simulink model "snb_a"  (R2012b)
settings: Solver=FixedStepDiscrete  SolverMode=SingleTasking  StartTime=0.0  StopTime=10000  RelTol=1e-3
undefined symbols (not defined in the file): Down, Up
libraries: xbsIndex_r4 x9360, casper_library_misc x16, casper_library_communications x8, xps_library x4, casper_library_delays x2
(part 5 of 71)

== system snb_a/coarse_delay3 ==
  note: new delay values/enables come aligned
      | with data, need to be one cycle before
      | so new delay value gets loaded at the
      | same time as data, so delay data path
      | by one cycle
  sync_in : Inport
  din0 : Inport  Port=2
  en : Inport  Port=3
  delay_val0 : Inport  Port=4
  load_val0 : Inport  Port=5
  Concat4 : xbsIndex_r4/Concat  num_inputs=8  dbl_ovrd=off  block_type=concat
  Delay36 : xbsIndex_r4/Delay  rst=off  infoeditControl=Selection of Reset will increase slice count due to use of real FFs and instead of SRLs  en=off  latency=1  dbl_ovrd=off  reg_retiming=on  block_type=delay
  Delay37 : xbsIndex_r4/Delay  rst=off  infoeditControl=Selection of Reset will increase slice count due to use of real FFs and instead of SRLs  en=off  latency=1  dbl_ovrd=off  reg_retiming=on  block_type=delay
  Delay38 : xbsIndex_r4/Delay  rst=off  infoeditControl=Selection of Reset will increase slice count due to use of real FFs and instead of SRLs  en=off  latency=1  dbl_ovrd=off  reg_retiming=on  block_type=delay
  Reinterpret{,1..7} (8 alike) : xbsIndex_r4/Reinterpret  force_arith_type=on  arith_type=Unsigned  force_bin_pt=on  bin_pt=0  block_type=reinterpret
  Terminator34 : Terminator
  Terminator38 : Terminator
  Terminator39 : Terminator
  bus_expand14 : Subsystem  AncestorBlock=casper_library_flow_control/bus_expand  mask(bus_expand){mode=divisions of arbitrary size, outputNum=1, outputWidth=[16+15 16 16 16], outputBinaryPt=[16 15 15 15], outputArithmeticType=[0 1 1 1], show_format=off, outputToWorkspace=off, variablePrefix=out, outputToModelAsWell=on}
      mask prompts: outputNum "Number of outputs:"; outputWidth "Output width [msb ... lsb]:"; outputBinaryPt "Output binary point position [msb ... lsb]:"; outputArithmeticType "Output arithmetic type (ufix=0, fix=1, bool=2) [msb ... lsb]:"; show_format "Print format string?"; outputToWorkspace "Output to workspace?"; variablePrefix "Variable name prefix:"; outputToModelAsWell "Output to model as well?"
      mask help:
      | Expands a 'bus' made using a bus_create or Xilinx
      | concat block.
      | The input will be divided into the specified number
      | of outputs with the specified arithmetic types.
      | Divisions are made from most significant bit.
      mask init: same as snb_a/bus_expand10
      settings: AttributesFormatString=4 outputs
      mask TypeOptions mode: divisions of equal size | divisions of arbitrary size
      mask Callback mode: bus_expand_callback();
      mask Callback outputWidth: bus_expand_callback();
      mask Callback outputToWorkspace: bus_expand_callback();
  bus_expand7 : Subsystem  AncestorBlock=casper_library_flow_control/bus_expand  mask(bus_expand){mode=divisions of equal size, outputNum=8, outputWidth=10, outputBinaryPt=9, outputArithmeticType=1, show_format=off, outputToWorkspace=off, variablePrefix=out, outputToModelAsWell=on}
      mask prompts: outputNum "Number of outputs:"; outputWidth "Output width:"; outputBinaryPt "Output binary point position:"; outputArithmeticType "Output arithmetic type (ufix=0, fix=1, bool=2):"; show_format "Print format string?"; outputToWorkspace "Output to workspace?"; variablePrefix "Variable name prefix:"; outputToModelAsWell "Output to model as well?"
      mask help:
      | Expands a 'bus' made using a bus_create or Xilinx
      | concat block.
      | The input will be divided into the specified number
      | of outputs with the specified arithmetic types.
      | Divisions are made from most significant bit.
      mask init: same as snb_a/bus_expand10
      settings: AttributesFormatString=8 outputs
      mask TypeOptions mode: divisions of equal size | divisions of arbitrary size
      mask Callback mode: bus_expand_callback();
      mask Callback outputWidth: bus_expand_callback();
      mask Callback outputToWorkspace: bus_expand_callback();
  delay_gen0 : Subsystem  mask{n_bits_fft_words=10, n_bits_streams=3, n_bits_fft=12, n_bits_data=10}
      mask prompts: n_bits_fft_words "FFT size (2^? data words)"; n_bits_streams "parallel data streams (2^?)"; n_bits_fft "effective FFT size (2^? bins)"; n_bits_data "data bit width"
  delay_wideband_prog0 : Subsystem  AncestorBlock=casper_library_delays/delay_wideband_prog  mask(delay_wideband_prog){max_delay=8192, n_inputs_bits=3, bram_latency=2, bram_type=Dual Port, async=on}
      mask prompts: max_delay "Max Delay (Sample Clks)"; n_inputs_bits "Number of Simultaneous Inputs(2^?)"; bram_latency "BRAM Latency"; bram_type "Select type of BRAM"; async "asynchronous operation"
      mask init:
      | delay_wideband_prog_init(gcb,...
      |     'max_delay',max_delay,...
      |     'n_inputs_bits',n_inputs_bits,...
      |     'bram_latency',bram_latency,...
      |     'bram_type',bram_type, ...
      |     'async', async);
      mask TypeOptions bram_type: Single Port | Dual Port
  sync_out : Outport
  dout0 : Outport  Port=2
  dvalid : Outport  Port=3
  wires:
  Reinterpret7/1 -> Concat4/8
  Reinterpret6/1 -> Concat4/7
  Reinterpret4/1 -> Concat4/5
  Reinterpret5/1 -> Concat4/6
  Reinterpret3/1 -> Concat4/4
  Reinterpret2/1 -> Concat4/3
  Reinterpret1/1 -> Concat4/2
  Reinterpret/1 -> Concat4/1
  delay_gen0/6(slope) -> Terminator39/1
  delay_gen0/5(initial_phase) -> Terminator38/1
  delay_gen0/3(idx_out) -> Terminator34/1
  din0/1 -> delay_gen0/2(din)
  bus_expand14/4(lsb_out1) -> delay_gen0/7(d/dt_phase)
  bus_expand14/3(out2) -> delay_gen0/6(phase)
  bus_expand14/2(out3) -> delay_gen0/5(d/dt_delay)
  bus_expand14/1(msb_out4) -> delay_gen0/4(delay)
  sync_in/1 -> delay_gen0/1(sync_in)
  delay_gen0/4(dvalid) -> Delay37/1
  delay_gen0/1(sync_out) -> Delay36/1
  delay_gen0/2(dout) -> Delay38/1
  delay_wideband_prog0/10(dvalid) -> dvalid/1
  bus_expand7/8(lsb_out1) -> delay_wideband_prog0/11(data_in7)
  bus_expand7/7(out2) -> delay_wideband_prog0/10(data_in6)
  bus_expand7/6(out3) -> delay_wideband_prog0/9(data_in5)
  bus_expand7/5(out4) -> delay_wideband_prog0/8(data_in4)
  bus_expand7/4(out5) -> delay_wideband_prog0/7(data_in3)
  bus_expand7/3(out6) -> delay_wideband_prog0/6(data_in2)
  bus_expand7/2(out7) -> delay_wideband_prog0/5(data_in1)
  bus_expand7/1(msb_out8) -> delay_wideband_prog0/4(data_in0)
  delay_gen0/8(new_value) -> delay_wideband_prog0/3(ld_delay)
  delay_gen0/7(coarse_delay) -> delay_wideband_prog0/2(delay)
  en/1 -> delay_gen0/3(en)
  load_val0/1 -> delay_gen0/8(ld)
  delay_val0/1 -> bus_expand14/1(bus_in)
  delay_wideband_prog0/1(sync_out) -> sync_out/1
  Delay38/1 -> bus_expand7/1(bus_in)
  delay_wideband_prog0/9(data_out7) -> Reinterpret7/1
  Delay36/1 -> delay_wideband_prog0/1(sync)
  delay_wideband_prog0/5(data_out3) -> Reinterpret3/1
  delay_wideband_prog0/4(data_out2) -> Reinterpret2/1
  Delay37/1 -> delay_wideband_prog0/12(en)
  Concat4/1 -> dout0/1
  delay_wideband_prog0/7(data_out5) -> Reinterpret5/1
  delay_wideband_prog0/8(data_out6) -> Reinterpret6/1
  delay_wideband_prog0/3(data_out1) -> Reinterpret1/1
  delay_wideband_prog0/6(data_out4) -> Reinterpret4/1
  delay_wideband_prog0/2(data_out0) -> Reinterpret/1

== system snb_a/control ==
  convert1_{1..21} (21 alike) : DataTypeConversion  OutDataTypeStr=fixdt('ufix1_En0')  LockScale=on
  convert2_{1..21} (21 alike) : DataTypeConversion  OutDataTypeStr=fixdt('ufix1_En0')  ConvertRealWorld=Stored Integer (SI)  LockScale=on
  gain_1 : Gain  Gain=1048576
  gain_10 : Gain  Gain=2048
  gain_11 : Gain  Gain=1024
  gain_12 : Gain  Gain=512
  gain_13 : Gain  Gain=256
  gain_14 : Gain  Gain=128
  gain_15 : Gain  Gain=64
  gain_16 : Gain  Gain=32
  gain_17 : Gain  Gain=16
  gain_18 : Gain  Gain=8
  gain_19 : Gain  Gain=4
  gain_2 : Gain  Gain=524288
  gain_20 : Gain  Gain=2
  gain_21 : Gain
  gain_3 : Gain  Gain=262144
  gain_4 : Gain  Gain=131072
  gain_5 : Gain  Gain=65536
  gain_6 : Gain  Gain=32768
  gain_7 : Gain  Gain=16384
  gain_8 : Gain  Gain=8192
  gain_9 : Gain  Gain=4096
  io_delay : xbsIndex_r4/Delay  rst=off  infoeditControl=Selection of Reset will increase slice count due to use of real FFs and instead of SRLs  en=off  latency=1  dbl_ovrd=off  reg_retiming=on  block_type=delay
  sim_{1..21} (21 alike) : Constant  Value=0
  sim_add : Sum  Inputs=+++++++++++++++++++++  OutDataTypeStr=uint32
  slice_adc_bad_clr : xbsIndex_r4/Slice  nbits=1  boolean_output=on  mode=Lower Bit Location + Width  bit1=0  base1=MSB of Input  bit0=15  base0=LSB of Input  dbl_ovrd=off  block_type=slice
  slice_adc_protect_disable : xbsIndex_r4/Slice  nbits=1  boolean_output=on  mode=Lower Bit Location + Width  bit1=0  base1=MSB of Input  bit0=14  base0=LSB of Input  dbl_ovrd=off  block_type=slice
  slice_arm : xbsIndex_r4/Slice  nbits=1  boolean_output=on  mode=Lower Bit Location + Width  bit1=0  base1=MSB of Input  bit0=19  base0=LSB of Input  dbl_ovrd=off  block_type=slice
  slice_cnt_rst : xbsIndex_r4/Slice  nbits=1  boolean_output=on  mode=Lower Bit Location + Width  bit1=0  base1=MSB of Input  bit0=8  base0=LSB of Input  dbl_ovrd=off  block_type=slice
  slice_gbe_cnt_rst : xbsIndex_r4/Slice  nbits=1  boolean_output=on  mode=Lower Bit Location + Width  bit1=0  base1=MSB of Input  bit0=7  base0=LSB of Input  dbl_ovrd=off  block_type=slice
  slice_gbe_rst : xbsIndex_r4/Slice  nbits=1  boolean_output=on  mode=Lower Bit Location + Width  bit1=0  base1=MSB of Input  bit0=17  base0=LSB of Input  dbl_ovrd=off  block_type=slice
  slice_gbe_txen : xbsIndex_r4/Slice  nbits=1  boolean_output=on  mode=Lower Bit Location + Width  bit1=0  base1=MSB of Input  bit0=16  base0=LSB of Input  dbl_ovrd=off  block_type=slice
  slice_snapcoarse_arm : xbsIndex_r4/Slice  nbits=1  boolean_output=on  mode=Lower Bit Location + Width  bit1=0  base1=MSB of Input  bit0=5  base0=LSB of Input  dbl_ovrd=off  block_type=slice
  slice_snappfb_arm : xbsIndex_r4/Slice  nbits=1  boolean_output=on  mode=Lower Bit Location + Width  bit1=0  base1=MSB of Input  bit0=4  base0=LSB of Input  dbl_ovrd=off  block_type=slice
  slice_snappfb_dsel : xbsIndex_r4/Slice  nbits=1  boolean_output=on  mode=Lower Bit Location + Width  bit1=0  base1=MSB of Input  bit0=3  base0=LSB of Input  dbl_ovrd=off  block_type=slice
  slice_snapquant_arm : xbsIndex_r4/Slice  nbits=1  boolean_output=on  mode=Lower Bit Location + Width  bit1=0  base1=MSB of Input  bit0=2  base0=LSB of Input  dbl_ovrd=off  block_type=slice
  slice_status_clr : xbsIndex_r4/Slice  nbits=1  boolean_output=on  mode=Lower Bit Location + Width  bit1=0  base1=MSB of Input  bit0=18  base0=LSB of Input  dbl_ovrd=off  block_type=slice
  slice_sys_rst : xbsIndex_r4/Slice  nbits=1  boolean_output=on  mode=Lower Bit Location + Width  bit1=0  base1=MSB of Input  bit0=20  base0=LSB of Input  dbl_ovrd=off  block_type=slice
  slice_tvg_adc : xbsIndex_r4/Slice  nbits=1  boolean_output=on  mode=Lower Bit Location + Width  bit1=0  base1=MSB of Input  bit0=9  base0=LSB of Input  dbl_ovrd=off  block_type=slice
  slice_tvg_ct : xbsIndex_r4/Slice  nbits=1  boolean_output=on  mode=Lower Bit Location + Width  bit1=0  base1=MSB of Input  bit0=12  base0=LSB of Input  dbl_ovrd=off  block_type=slice
  slice_tvg_d80 : xbsIndex_r4/Slice  nbits=1  boolean_output=on  mode=Lower Bit Location + Width  bit1=0  base1=MSB of Input  bit0=1  base0=LSB of Input  dbl_ovrd=off  block_type=slice
  slice_tvg_en : xbsIndex_r4/Slice  nbits=1  boolean_output=on  mode=Lower Bit Location + Width  bit1=0  base1=MSB of Input  bit0=13  base0=LSB of Input  dbl_ovrd=off  block_type=slice
  slice_tvg_fdfs : xbsIndex_r4/Slice  nbits=1  boolean_output=on  mode=Lower Bit Location + Width  bit1=0  base1=MSB of Input  bit0=10  base0=LSB of Input  dbl_ovrd=off  block_type=slice
  slice_tvg_packetiser : xbsIndex_r4/Slice  nbits=1  boolean_output=on  mode=Lower Bit Location + Width  bit1=0  base1=MSB of Input  bit0=11  base0=LSB of Input  dbl_ovrd=off  block_type=slice
  slice_unpack_cnt_rst : xbsIndex_r4/Slice  nbits=1  boolean_output=on  mode=Lower Bit Location + Width  bit1=0  base1=MSB of Input  bit0=6  base0=LSB of Input  dbl_ovrd=off  block_type=slice
  slice_wintime_snap_wesel : xbsIndex_r4/Slice  nbits=1  boolean_output=on  mode=Lower Bit Location + Width  bit1=0  base1=MSB of Input  bit0=0  base0=LSB of Input  dbl_ovrd=off  block_type=slice
  snb_a_control_user_data_out : xbsIndex_r4/Gateway In  gui_display_data_type=Fixed-point  arith_type=Unsigned  n_bits=32  bin_pt=0  preci_type=Single  exp_width=8  frac_width=24  quantization="Round  (unbiased: +/- Inf)"  overflow=Saturate  period=1  dbl_ovrd=off  timing_constraint=None  locs_specified=off  LOCs={}  UseAsADC=off  ADCChannel='1'  inherit_from_input=off  hdl_port=on  block_type=gatewayin
  in_sys_rst : Outport
  in_arm : Outport  Port=2
  in_status_clr : Outport  Port=3
  in_gbe_rst : Outport  Port=4
  in_gbe_txen : Outport  Port=5
  in_adc_bad_clr : Outport  Port=6
  in_adc_protect_disable : Outport  Port=7
  in_tvg_en : Outport  Port=8
  in_tvg_ct : Outport  Port=9
  in_tvg_packetiser : Outport  Port=10
  in_tvg_fdfs : Outport  Port=11
  in_tvg_adc : Outport  Port=12
  in_cnt_rst : Outport  Port=13
  in_gbe_cnt_rst : Outport  Port=14
  in_unpack_cnt_rst : Outport  Port=15
  in_snapcoarse_arm : Outport  Port=16
  in_snappfb_arm : Outport  Port=17
  in_snappfb_dsel : Outport  Port=18
  in_snapquant_arm : Outport  Port=19
  in_tvg_d80 : Outport  Port=20
  in_wintime_snap_wesel : Outport  Port=21
  wires:
  snb_a_control_user_data_out/1 -> io_delay/1
  sim_add/1 -> snb_a_control_user_data_out/1
  sim_1/1 -> convert1_1/1
  convert1_1/1 -> convert2_1/1
  convert2_1/1 -> gain_1/1
  gain_1/1 -> sim_add/1
  io_delay/1 -> slice_sys_rst/1, slice_arm/1, slice_status_clr/1, slice_gbe_rst/1, slice_gbe_txen/1, slice_adc_bad_clr/1, slice_adc_protect_disable/1, slice_tvg_en/1, slice_tvg_ct/1, slice_tvg_packetiser/1, slice_tvg_fdfs/1, slice_tvg_adc/1, slice_cnt_rst/1, slice_gbe_cnt_rst/1, slice_unpack_cnt_rst/1, slice_snapcoarse_arm/1, slice_snappfb_arm/1, slice_snappfb_dsel/1, slice_snapquant_arm/1, slice_tvg_d80/1, slice_wintime_snap_wesel/1
  slice_sys_rst/1 -> in_sys_rst/1
  sim_2/1 -> convert1_2/1
  convert1_2/1 -> convert2_2/1
  convert2_2/1 -> gain_2/1
  gain_2/1 -> sim_add/2
  slice_arm/1 -> in_arm/1
  sim_3/1 -> convert1_3/1
  convert1_3/1 -> convert2_3/1
  convert2_3/1 -> gain_3/1
  gain_3/1 -> sim_add/3
  slice_status_clr/1 -> in_status_clr/1
  sim_4/1 -> convert1_4/1
  convert1_4/1 -> convert2_4/1
  convert2_4/1 -> gain_4/1
  gain_4/1 -> sim_add/4
  slice_gbe_rst/1 -> in_gbe_rst/1
  sim_5/1 -> convert1_5/1
  convert1_5/1 -> convert2_5/1
  convert2_5/1 -> gain_5/1
  gain_5/1 -> sim_add/5
  slice_gbe_txen/1 -> in_gbe_txen/1
  sim_6/1 -> convert1_6/1
  convert1_6/1 -> convert2_6/1
  convert2_6/1 -> gain_6/1
  gain_6/1 -> sim_add/6
  slice_adc_bad_clr/1 -> in_adc_bad_clr/1
  sim_7/1 -> convert1_7/1
  convert1_7/1 -> convert2_7/1
  convert2_7/1 -> gain_7/1
  gain_7/1 -> sim_add/7
  slice_adc_protect_disable/1 -> in_adc_protect_disable/1
  sim_8/1 -> convert1_8/1
  convert1_8/1 -> convert2_8/1
  convert2_8/1 -> gain_8/1
  gain_8/1 -> sim_add/8
  slice_tvg_en/1 -> in_tvg_en/1
  sim_9/1 -> convert1_9/1
  convert1_9/1 -> convert2_9/1
  convert2_9/1 -> gain_9/1
  gain_9/1 -> sim_add/9
  slice_tvg_ct/1 -> in_tvg_ct/1
  sim_10/1 -> convert1_10/1
  convert1_10/1 -> convert2_10/1
  convert2_10/1 -> gain_10/1
  gain_10/1 -> sim_add/10
  slice_tvg_packetiser/1 -> in_tvg_packetiser/1
  sim_11/1 -> convert1_11/1
  convert1_11/1 -> convert2_11/1
  convert2_11/1 -> gain_11/1
  gain_11/1 -> sim_add/11
  slice_tvg_fdfs/1 -> in_tvg_fdfs/1
  sim_12/1 -> convert1_12/1
  convert1_12/1 -> convert2_12/1
  convert2_12/1 -> gain_12/1
  gain_12/1 -> sim_add/12
  slice_tvg_adc/1 -> in_tvg_adc/1
  sim_13/1 -> convert1_13/1
  convert1_13/1 -> convert2_13/1
  convert2_13/1 -> gain_13/1
  gain_13/1 -> sim_add/13
  slice_cnt_rst/1 -> in_cnt_rst/1
  sim_14/1 -> convert1_14/1
  convert1_14/1 -> convert2_14/1
  convert2_14/1 -> gain_14/1
  gain_14/1 -> sim_add/14
  slice_gbe_cnt_rst/1 -> in_gbe_cnt_rst/1
  sim_15/1 -> convert1_15/1
  convert1_15/1 -> convert2_15/1
  convert2_15/1 -> gain_15/1
  gain_15/1 -> sim_add/15
  slice_unpack_cnt_rst/1 -> in_unpack_cnt_rst/1
  sim_16/1 -> convert1_16/1
  convert1_16/1 -> convert2_16/1
  convert2_16/1 -> gain_16/1
  gain_16/1 -> sim_add/16
  slice_snapcoarse_arm/1 -> in_snapcoarse_arm/1
  sim_17/1 -> convert1_17/1
  convert1_17/1 -> convert2_17/1
  convert2_17/1 -> gain_17/1
  gain_17/1 -> sim_add/17
  slice_snappfb_arm/1 -> in_snappfb_arm/1
  sim_18/1 -> convert1_18/1
  convert1_18/1 -> convert2_18/1
  convert2_18/1 -> gain_18/1
  gain_18/1 -> sim_add/18
  slice_snappfb_dsel/1 -> in_snappfb_dsel/1
  sim_19/1 -> convert1_19/1
  convert1_19/1 -> convert2_19/1
  convert2_19/1 -> gain_19/1
  gain_19/1 -> sim_add/19
  slice_snapquant_arm/1 -> in_snapquant_arm/1
  sim_20/1 -> convert1_20/1
  convert1_20/1 -> convert2_20/1
  convert2_20/1 -> gain_20/1
  gain_20/1 -> sim_add/20
  slice_tvg_d80/1 -> in_tvg_d80/1
  sim_21/1 -> convert1_21/1
  convert1_21/1 -> convert2_21/1
  convert2_21/1 -> gain_21/1
  gain_21/1 -> sim_add/21
  slice_wintime_snap_wesel/1 -> in_wintime_snap_wesel/1

== system snb_a/ct ==
  sync : Inport
  valid : Inport  Port=2
  din0 : Inport  Port=3
  din1 : Inport  Port=4
  Concat : xbsIndex_r4/Concat  num_inputs=2  dbl_ovrd=off  block_type=concat
  Concat1 : xbsIndex_r4/Concat  num_inputs=2  dbl_ovrd=off  block_type=concat
  Delay{1,3..7,9..12,14..20} (17 alike) : xbsIndex_r4/Delay  rst=off  infoeditControl=Selection of Reset will increase slice count due to use of real FFs and instead of SRLs  en=off  latency=1  dbl_ovrd=off  reg_retiming=on  block_type=delay
  Delay2 : xbsIndex_r4/Delay  rst=off  infoeditControl=Selection of Reset will increase slice count due to use of real FFs and instead of SRLs  en=off  latency=1  dbl_ovrd=off  reg_retiming=off  block_type=delay
  Gateway Out{,1..9} (10 alike) : xbsIndex_r4/Gateway Out  inherit_from_input=off  hdl_port=on  timing_constraint=None  locs_specified=off  LOCs={}  UseAsDAC=off  DACChannel='1'  block_type=gatewayout
  Logical : xbsIndex_r4/Logical  logical_function=OR  inputs=2  en=off  latency=0  precision=Full  arith_type=Unsigned  n_bits=16  bin_pt=0  align_bp=on  dbl_ovrd=off  block_type=logical
  Scope : Scope  NumInputPorts=10
      settings: YMin=-1~0~0~-1~0~0~-5~-5~-5~-5  YMax=1~1~70000~1~1~70000~5~5~5~5  SaveName=ScopeData9
  Slice3 : xbsIndex_r4/Slice  nbits=1  boolean_output=on  mode=Upper Bit Location + Width  bit1=0  base1=MSB of Input  bit0=0  base0=LSB of Input  dbl_ovrd=off  block_type=slice
  Slice4 : xbsIndex_r4/Slice  nbits=16  boolean_output=off  mode=Lower Bit Location + Width  bit1=0  base1=MSB of Input  bit0=0  base0=LSB of Input  dbl_ovrd=off  block_type=slice
  Slice5 : xbsIndex_r4/Slice  nbits=16  boolean_output=off  mode=Lower Bit Location + Width  bit1=0  base1=MSB of Input  bit0=0  base0=LSB of Input  dbl_ovrd=off  block_type=slice
  Terminator : Terminator
  bus_expand : Subsystem  AncestorBlock=casper_library_flow_control/bus_expand  mask(bus_expand){mode=divisions of equal size, outputNum=4, outputWidth=64, outputBinaryPt=0, outputArithmeticType=0, show_format=off, outputToWorkspace=off, variablePrefix=out, outputToModelAsWell=on}
      mask prompts: outputNum "Number of outputs:"; outputWidth "Output width:"; outputBinaryPt "Output binary point position:"; outputArithmeticType "Output arithmetic type (ufix=0, fix=1, bool=2):"; show_format "Print format string?"; outputToWorkspace "Output to workspace?"; variablePrefix "Variable name prefix:"; outputToModelAsWell "Output to model as well?"
      mask help:
      | Expands a 'bus' made using a bus_create or Xilinx
      | concat block.
      | The input will be divided into the specified number
      | of outputs with the specified arithmetic types.
      | Divisions are made from most significant bit.
      mask init: same as snb_a/bus_expand10
      settings: AttributesFormatString=4 outputs
      mask TypeOptions mode: divisions of equal size | divisions of arbitrary size
      mask Callback mode: bus_expand_callback();
      mask Callback outputWidth: bus_expand_callback();
      mask Callback outputToWorkspace: bus_expand_callback();
  concat0 : xbsIndex_r4/Concat  num_inputs=2  dbl_ovrd=off  block_type=concat
  concat1 : xbsIndex_r4/Concat  num_inputs=2  dbl_ovrd=off  block_type=concat
  counter : xbsIndex_r4/Counter  cnt_type=Free Running  cnt_to=Inf  operation=Up  start_count=0  cnt_by_val=1  arith_type=Unsigned  n_bits=1  bin_pt=0  load_pin=off  rst=on  en=on  explicit_period=on  period=1  dbl_ovrd=off  use_behavioral_HDL=off  implementation=Fabric  block_type=counter
  ct0 : Subsystem  mask{idepth=input_bits, odepth=output_bits, which_qdr=qdr0, swap_input=no, output_order=interleaved, step_bits=xeng_bits, custom_map=[0 2 4 6 8 10 12 14 1 3 5 7 9 11 13 15]}
      mask prompts: idepth "Input vector length (2^?)"; odepth "Output vector length (2^?)"; which_qdr "QDR SRAM chip"; swap_input "Swap input halves?"; output_order "Output column order"; step_bits "Interleave step (2^?)"; custom_map "Custom map"
      mask help:
      | Writes vectors in as rows in matrix and reads
      | out columns. Order in which columns read out
      | determined by 'Output column order' parameter.
      mask init:
      | if strcmp(output_order, 'interleaved') == 1 && (step_bits > idepth-1) ,
      |     disp('Can''t make step size bigger than (output vector bit size - 1)')
      |     return;
      | end    
      | 
      | if strcmp(output_order, 'custom') && (...
      |         length(unique(custom_map)) ~= 2^idepth ||...
      |         ~isempty(find(custom_map < 0)) || ...
      |         ~isempty(find(custom_map > (2^idepth)-1))),
      |     disp('Custom map elements must be unique in range 0->2^(input vector)-1');
      |     return;
      | end
      | 
      | % set up output order (in order, interleaved, or custom)
      | map = '[0:(2^idepth)-1]';
      | if strcmp(swap_input, 'yes'),
      |     %map = [map((length(map)/2)+1:end), map(1:length(map)/2)];
      |     map = '[2^(idepth-1):(2^idepth)-1, 0:2^(idepth-1)-1]';
      | end
      | if strcmp(output_order, 'interleaved'),
      |     map = ['reshape(reshape(', map,', 2^(idepth-step_bits), 2^step_bits)'', 1, 2^idepth)'];  
      |     
      | %    index = zeros(1, 2^idepth);
      | %    step_size = 2^(idepth-step_bits);
      | %    for ctr = 0:(2^step_bits)-1,
      | %        start = (ctr * step_size) + 1;
      | %        finish = start + step_size - 1;
      | %        index(start:finish) = ctr+1 : 2^step_bits : 2^idepth;
      | %    end
      | %    map = map(index);
      | %    clear index;
      | elseif strcmp(output_order, 'custom'),
      |     map = custom_map;
      | end
      | 
      | %generate map so that two samples from same position in 
      | %subsequent input vectors are written into same address
      | map = ['reshape([', map,'; 2^idepth+', map, '], 1 ,2^(idepth+1))'];
      | 
      | set_param([gcb, '/reorder'], 'map', map);
      | set_param([gcb, '/qdr'], 'which_qdr', which_qdr);
      mask TypeOptions which_qdr: qdr0 | qdr1 | qdr2 | qdr3
      mask TypeOptions swap_input: no | yes
      mask TypeOptions output_order: in order | interleaved | custom
  ct1 : Subsystem  mask{idepth=input_bits, odepth=output_bits, which_qdr=qdr1, swap_input=no, output_order=interleaved, step_bits=xeng_bits, custom_map=[0 2 4 6 8 10 12 14 1 3 5 7 9 11 13 15]}
      mask prompts: idepth "Input vector length (2^?)"; odepth "Output vector length (2^?)"; which_qdr "QDR SRAM chip"; swap_input "Swap input halves?"; output_order "Output column order"; step_bits "Interleave step (2^?)"; custom_map "Custom map"
      mask help:
      | Writes vectors in as rows in matrix and reads
      | out columns. Order in which columns read out
      | determined by 'Output column order' parameter.
      mask init: same as snb_a/ct/ct0
      mask TypeOptions which_qdr: qdr0 | qdr1 | qdr2 | qdr3
      mask TypeOptions swap_input: no | yes
      mask TypeOptions output_order: in order | interleaved | custom
  logical1 : xbsIndex_r4/Logical  logical_function=AND  inputs=2  en=off  latency=1  precision=Full  arith_type=Unsigned  n_bits=16  bin_pt=0  align_bp=on  dbl_ovrd=off  block_type=logical
  munge : Subsystem  AncestorBlock=casper_library_flow_control/munge  mask(munge){divisions=16, div_size=repmat(16, 1, 16), order=[0 4 8 12 1 5 9 13 2 6 10 14 3 7 11 15], arith_type_out=Unsigned, bin_pt_out=0}
      mask prompts: divisions "Number of divisions"; div_size "Division size (bits)"; order "Division packing order"; arith_type_out "Output arithmetic type"; bin_pt_out "Output binary point"
      mask help: Splits an input bus into the specified number of divisions and then recombines them in the order specified (most significant division = 0,least = number divisions-1)
      mask init:
      | munge_init(gcb, ...
      |     'divisions', divisions, ...
      |     'div_size', div_size, ...
      |     'order', order, ...
      |     'arith_type_out', arith_type_out, ...
      |     'bin_pt_out', bin_pt_out);
      settings: AttributesFormatString=|
      | split:[16 16 16 16 16 16 16 16 16 16 16 16 16 16 16 16]
      | join:[0 4 8 12 1 5 9 13 2 6 10 14 3 7 11 15]
      | Unsigned [256,0]
      mask TypeOptions arith_type_out: Unsigned | Signed  (2's comp) | Floating-point
  parity_check0 : Subsystem
  parity_check1 : Subsystem
  parity_generation0 : Subsystem
  parity_generation1 : Subsystem
  pipeline : Subsystem  AncestorBlock=casper_library_delays/pipeline  mask(pipeline){latency=3}
      mask help:
      | An explicitly laid-out delay line to avoid mapping to SRL16s
      | for use in pipelining to help achieve timing closure.
      mask init:
      | pipeline_init(gcb,'latency',latency);
      settings: AttributesFormatString=Latency = %<latency>
      mask Display:
      | port_label('input', 1, 'd');
      | port_label('output', 1, 'q');
      | disp(['Z^-', num2str(latency)]);
  pipeline1 : Subsystem  AncestorBlock=casper_library_delays/pipeline  mask(pipeline){latency=3}
      mask help:
      | An explicitly laid-out delay line to avoid mapping to SRL16s
      | for use in pipelining to help achieve timing closure.
      mask init:
      | pipeline_init(gcb,'latency',latency);
      settings: AttributesFormatString=Latency = %<latency>
      mask Display:
      | port_label('input', 1, 'd');
      | port_label('output', 1, 'q');
      | disp(['Z^-', num2str(latency)]);
  pipeline10 : Subsystem  AncestorBlock=casper_library_delays/pipeline  mask(pipeline){latency=3}
      mask help:
      | An explicitly laid-out delay line to avoid mapping to SRL16s
      | for use in pipelining to help achieve timing closure.
      mask init:
      | pipeline_init(gcb,'latency',latency);
      settings: AttributesFormatString=Latency = %<latency>
      mask Display:
      | port_label('input', 1, 'd');
      | port_label('output', 1, 'q');
      | disp(['Z^-', num2str(latency)]);
  pipeline11 : Subsystem  AncestorBlock=casper_library_delays/pipeline  mask(pipeline){latency=3}
      mask help:
      | An explicitly laid-out delay line to avoid mapping to SRL16s
      | for use in pipelining to help achieve timing closure.
      mask init:
      | pipeline_init(gcb,'latency',latency);
      settings: AttributesFormatString=Latency = %<latency>
      mask Display:
      | port_label('input', 1, 'd');
      | port_label('output', 1, 'q');
      | disp(['Z^-', num2str(latency)]);
  pipeline12 : Subsystem  AncestorBlock=casper_library_delays/pipeline  mask(pipeline){latency=3}
      mask help:
      | An explicitly laid-out delay line to avoid mapping to SRL16s
      | for use in pipelining to help achieve timing closure.
      mask init:
      | pipeline_init(gcb,'latency',latency);
      settings: AttributesFormatString=Latency = %<latency>
      mask Display:
      | port_label('input', 1, 'd');
      | port_label('output', 1, 'q');
      | disp(['Z^-', num2str(latency)]);
  pipeline13 : Subsystem  AncestorBlock=casper_library_delays/pipeline  mask(pipeline){latency=3}
      mask help:
      | An explicitly laid-out delay line to avoid mapping to SRL16s
      | for use in pipelining to help achieve timing closure.
      mask init:
      | pipeline_init(gcb,'latency',latency);
      settings: AttributesFormatString=Latency = %<latency>
      mask Display:
      | port_label('input', 1, 'd');
      | port_label('output', 1, 'q');
      | disp(['Z^-', num2str(latency)]);
  pipeline2 : Subsystem  AncestorBlock=casper_library_delays/pipeline  mask(pipeline){latency=3}
      mask help:
      | An explicitly laid-out delay line to avoid mapping to SRL16s
      | for use in pipelining to help achieve timing closure.
      mask init:
      | pipeline_init(gcb,'latency',latency);
      settings: AttributesFormatString=Latency = %<latency>
      mask Display:
      | port_label('input', 1, 'd');
      | port_label('output', 1, 'q');
      | disp(['Z^-', num2str(latency)]);
  pipeline3 : Subsystem  AncestorBlock=casper_library_delays/pipeline  mask(pipeline){latency=3}
      mask help:
      | An explicitly laid-out delay line to avoid mapping to SRL16s
      | for use in pipelining to help achieve timing closure.
      mask init:
      | pipeline_init(gcb,'latency',latency);
      settings: AttributesFormatString=Latency = %<latency>
      mask Display:
      | port_label('input', 1, 'd');
      | port_label('output', 1, 'q');
      | disp(['Z^-', num2str(latency)]);
  pipeline4 : Subsystem  AncestorBlock=casper_library_delays/pipeline  mask(pipeline){latency=3}
      mask help:
      | An explicitly laid-out delay line to avoid mapping to SRL16s
      | for use in pipelining to help achieve timing closure.
      mask init:
      | pipeline_init(gcb,'latency',latency);
      settings: AttributesFormatString=Latency = %<latency>
      mask Display:
      | port_label('input', 1, 'd');
      | port_label('output', 1, 'q');
      | disp(['Z^-', num2str(latency)]);
  pipeline5 : Subsystem  AncestorBlock=casper_library_delays/pipeline  mask(pipeline){latency=3}
      mask help:
      | An explicitly laid-out delay line to avoid mapping to SRL16s
      | for use in pipelining to help achieve timing closure.
      mask init:
      | pipeline_init(gcb,'latency',latency);
      settings: AttributesFormatString=Latency = %<latency>
      mask Display:
      | port_label('input', 1, 'd');
      | port_label('output', 1, 'q');
      | disp(['Z^-', num2str(latency)]);
  pipeline6 : Subsystem  AncestorBlock=casper_library_delays/pipeline  mask(pipeline){latency=3}
      mask help:
      | An explicitly laid-out delay line to avoid mapping to SRL16s
      | for use in pipelining to help achieve timing closure.
      mask init:
      | pipeline_init(gcb,'latency',latency);
      settings: AttributesFormatString=Latency = %<latency>
      mask Display:
      | port_label('input', 1, 'd');
      | port_label('output', 1, 'q');
      | disp(['Z^-', num2str(latency)]);
  pipeline7 : Subsystem  AncestorBlock=casper_library_delays/pipeline  mask(pipeline){latency=3}
      mask help:
      | An explicitly laid-out delay line to avoid mapping to SRL16s
      | for use in pipelining to help achieve timing closure.
      mask init:
      | pipeline_init(gcb,'latency',latency);
      settings: AttributesFormatString=Latency = %<latency>
      mask Display:
      | port_label('input', 1, 'd');
      | port_label('output', 1, 'q');
      | disp(['Z^-', num2str(latency)]);
  pipeline8 : Subsystem  AncestorBlock=casper_library_delays/pipeline  mask(pipeline){latency=3}
      mask help:
      | An explicitly laid-out delay line to avoid mapping to SRL16s
      | for use in pipelining to help achieve timing closure.
      mask init:
      | pipeline_init(gcb,'latency',latency);
      settings: AttributesFormatString=Latency = %<latency>
      mask Display:
      | port_label('input', 1, 'd');
      | port_label('output', 1, 'q');
      | disp(['Z^-', num2str(latency)]);
  pipeline9 : Subsystem  AncestorBlock=casper_library_delays/pipeline  mask(pipeline){latency=3}
      mask help:
      | An explicitly laid-out delay line to avoid mapping to SRL16s
      | for use in pipelining to help achieve timing closure.
      mask init:
      | pipeline_init(gcb,'latency',latency);
      settings: AttributesFormatString=Latency = %<latency>
      mask Display:
      | port_label('input', 1, 'd');
      | port_label('output', 1, 'q');
      | disp(['Z^-', num2str(latency)]);
  register : xbsIndex_r4/Register  init=0  rst=off  en=on  dbl_ovrd=off  block_type=register
  sync_out : Outport
  dvalid : Outport  Port=2
  dout0 : Outport  Port=3
  dout1 : Outport  Port=4
  dout2 : Outport  Port=5
  dout3 : Outport  Port=6
  ct_err : Outport  Port=7
  parity_error : Outport  Port=8
  wires:
  parity_check1/3(dvalid) -> counter/2, Delay11/1, Delay6/1
  parity_check1/4(error) -> Concat1/2
  parity_check1/1(sync_out) -> counter/1, Delay10/1
  ct1/3(dv) -> pipeline12/1(d)
  ct1/2(q) -> pipeline11/1(d)
  ct1/1(sync_out) -> pipeline10/1(d)
  parity_check0/3(dvalid) -> Terminator/1, Delay9/1
  parity_check0/1(sync_out) -> Delay1/1
  Concat1/1 -> parity_error/1
  parity_check0/4(error) -> Concat1/1
  ct0/3(dv) -> pipeline8/1(d)
  ct0/1(sync_out) -> pipeline6/1(d)
  ct0/2(q) -> pipeline7/1(d)
  din1/1 -> parity_generation1/2(din)
  parity_generation1/3(dvalid) -> pipeline5/1(d)
  parity_generation1/2(dout) -> pipeline4/1(d)
  parity_generation1/1(sync_out) -> pipeline3/1(d)
  parity_generation0/3(dvalid) -> pipeline2/1(d)
  parity_generation0/1(sync_out) -> pipeline/1(d)
  din0/1 -> parity_generation0/2(din)
  sync/1 -> parity_generation0/1(sync_in), parity_generation1/1(sync_in)
  Delay12/1 -> Delay19/1
  Delay20/1 -> Gateway Out7/1
  Delay19/1 -> Gateway Out6/1
  Delay18/1 -> Slice5/1
  Delay17/1 -> Gateway Out4/1
  Delay16/1 -> Gateway Out3/1
  Delay15/1 -> Slice4/1
  Delay14/1 -> Gateway Out1/1
  Delay3/1 -> sync_out/1, Gateway Out8/1, Gateway Out/1, Logical/1
  counter/1 -> Delay12/1, Slice3/1
  Delay11/1 -> Delay17/1
  Delay10/1 -> Delay16/1
  Delay9/1 -> Delay14/1
  Slice5/1 -> Gateway Out5/1
  Slice4/1 -> Gateway Out2/1
  Gateway Out6/1 -> Scope/7
  Gateway Out4/1 -> Scope/5
  Gateway Out1/1 -> Scope/2
  Gateway Out9/1 -> Scope/10
  Gateway Out8/1 -> Scope/9
  Gateway Out3/1 -> Scope/4
  Gateway Out2/1 -> Scope/3
  Gateway Out/1 -> Scope/1
  Gateway Out5/1 -> Scope/6
  Gateway Out7/1 -> Scope/8
  Logical/1 -> dvalid/1, Gateway Out9/1
  logical1/1 -> Logical/2
  Slice3/1 -> Delay7/1
  Delay6/1 -> logical1/1, register/2
  Delay5/1 -> concat0/2, Delay18/1
  Delay4/1 -> concat0/1, Delay15/1
  Delay1/1 -> Delay3/1, Delay20/1
  Delay2/1 -> munge/1(din)
  parity_check0/2(dout) -> Delay4/1
  parity_check1/2(dout) -> Delay5/1
  Delay7/1 -> logical1/2
  bus_expand/4(lsb_out1) -> dout3/1
  bus_expand/3(out2) -> dout2/1
  bus_expand/2(out3) -> dout1/1
  bus_expand/1(msb_out4) -> dout0/1
  munge/1(dout) -> bus_expand/1(bus_in)
  concat1/1 -> Delay2/1
  register/1 -> concat1/1
  concat0/1 -> register/1, concat1/2
  ct0/4(qdr_error) -> pipeline9/1(d)
  valid/1 -> parity_generation0/3(en), parity_generation1/3(en)
  Concat/1 -> ct_err/1
  ct1/4(qdr_error) -> pipeline13/1(d)
  parity_generation0/2(dout) -> pipeline1/1(d)
  pipeline/1(q) -> ct0/1(sync)
  pipeline1/1(q) -> ct0/2(d)
  pipeline2/1(q) -> ct0/3(en)
  pipeline3/1(q) -> ct1/1(sync)
  pipeline4/1(q) -> ct1/2(d)
  pipeline5/1(q) -> ct1/3(en)
  pipeline6/1(q) -> parity_check0/1(sync_in)
  pipeline7/1(q) -> parity_check0/2(din)
  pipeline8/1(q) -> parity_check0/3(en)
  pipeline9/1(q) -> Concat/1
  pipeline10/1(q) -> parity_check1/1(sync_in)
  pipeline11/1(q) -> parity_check1/2(din)
  pipeline12/1(q) -> parity_check1/3(en)
  pipeline13/1(q) -> Concat/2

== system snb_a/ct_cnt ==
  out_validcnt : Inport
  out_synccnt : Inport  Port=2
  assert_synccnt : xbsIndex_r4/Assert  assert_type=on  type_source=Explicitly  gui_display_data_type=Fixed-point  arith_type=Unsigned  n_bits=16  bin_pt=0  preci_type=Single  exp_width=8  frac_width=24  assert_rate=off  rate_source=Explicitly  period=1  output_port=on  block_type=assert
  assert_validcnt : xbsIndex_r4/Assert  assert_type=on  type_source=Explicitly  gui_display_data_type=Fixed-point  arith_type=Unsigned  n_bits=16  bin_pt=0  preci_type=Single  exp_width=8  frac_width=24  assert_rate=off  rate_source=Explicitly  period=1  output_port=on  block_type=assert
  cast_gw : xbsIndex_r4/Convert  gui_display_data_type=Fixed-point  arith_type=Unsigned  n_bits=32  bin_pt=0  float_type=Single  exp_bits=8  fraction_bits=24  quantization=Truncate  overflow=Wrap  en=off  latency=0  dbl_ovrd=off  pipeline=off  block_type=convert
  concatenate : xbsIndex_r4/Concat  num_inputs=2  dbl_ovrd=off  block_type=concat
  io_delay : xbsIndex_r4/Delay  rst=off  infoeditControl=Selection of Reset will increase slice count due to use of real FFs and instead of SRLs  en=off  latency=0  dbl_ovrd=off  reg_retiming=on  block_type=delay
  reint1 : xbsIndex_r4/Reinterpret  force_arith_type=on  arith_type=Unsigned  force_bin_pt=on  bin_pt=0  block_type=reinterpret
  reint2 : xbsIndex_r4/Reinterpret  force_arith_type=on  arith_type=Unsigned  force_bin_pt=on  bin_pt=0  block_type=reinterpret
  sim_out : Terminator
  snb_a_ct_cnt_user_data_in : xbsIndex_r4/Gateway Out  inherit_from_input=off  hdl_port=on  timing_constraint=None  locs_specified=off  LOCs={}  UseAsDAC=off  DACChannel='1'  block_type=gatewayout
  wires:
  concatenate/1 -> io_delay/1
  io_delay/1 -> cast_gw/1
  cast_gw/1 -> snb_a_ct_cnt_user_data_in/1
  snb_a_ct_cnt_user_data_in/1 -> sim_out/1
  out_validcnt/1 -> assert_validcnt/1
  assert_validcnt/1 -> reint1/1
  reint1/1 -> concatenate/1
  out_synccnt/1 -> assert_synccnt/1
  assert_synccnt/1 -> reint2/1
  reint2/1 -> concatenate/2

== system snb_a/ct_errcnt ==
  out_errcnt0 : Inport
  out_parerrcnt0 : Inport  Port=2
  out_errcnt1 : Inport  Port=3
  out_parerrcnt1 : Inport  Port=4
  assert_errcnt0 : xbsIndex_r4/Assert  assert_type=on  type_source=Explicitly  gui_display_data_type=Fixed-point  arith_type=Unsigned  n_bits=8  bin_pt=0  preci_type=Single  exp_width=8  frac_width=24  assert_rate=off  rate_source=Explicitly  period=1  output_port=on  block_type=assert
  assert_errcnt1 : xbsIndex_r4/Assert  assert_type=on  type_source=Explicitly  gui_display_data_type=Fixed-point  arith_type=Unsigned  n_bits=8  bin_pt=0  preci_type=Single  exp_width=8  frac_width=24  assert_rate=off  rate_source=Explicitly  period=1  output_port=on  block_type=assert
  assert_parerrcnt0 : xbsIndex_r4/Assert  assert_type=on  type_source=Explicitly  gui_display_data_type=Fixed-point  arith_type=Unsigned  n_bits=8  bin_pt=0  preci_type=Single  exp_width=8  frac_width=24  assert_rate=off  rate_source=Explicitly  period=1  output_port=on  block_type=assert
  assert_parerrcnt1 : xbsIndex_r4/Assert  assert_type=on  type_source=Explicitly  gui_display_data_type=Fixed-point  arith_type=Unsigned  n_bits=8  bin_pt=0  preci_type=Single  exp_width=8  frac_width=24  assert_rate=off  rate_source=Explicitly  period=1  output_port=on  block_type=assert
  cast_gw : xbsIndex_r4/Convert  gui_display_data_type=Fixed-point  arith_type=Unsigned  n_bits=32  bin_pt=0  float_type=Single  exp_bits=8  fraction_bits=24  quantization=Truncate  overflow=Wrap  en=off  latency=0  dbl_ovrd=off  pipeline=off  block_type=convert
  concatenate : xbsIndex_r4/Concat  num_inputs=4  dbl_ovrd=off  block_type=concat
  io_delay : xbsIndex_r4/Delay  rst=off  infoeditControl=Selection of Reset will increase slice count due to use of real FFs and instead of SRLs  en=off  latency=0  dbl_ovrd=off  reg_retiming=on  block_type=delay
  reint{1..4} (4 alike) : xbsIndex_r4/Reinterpret  force_arith_type=on  arith_type=Unsigned  force_bin_pt=on  bin_pt=0  block_type=reinterpret
  sim_out : Terminator
  snb_a_ct_errcnt_user_data_in : xbsIndex_r4/Gateway Out  inherit_from_input=off  hdl_port=on  timing_constraint=None  locs_specified=off  LOCs={}  UseAsDAC=off  DACChannel='1'  block_type=gatewayout
  wires:
  concatenate/1 -> io_delay/1
  io_delay/1 -> cast_gw/1
  cast_gw/1 -> snb_a_ct_errcnt_user_data_in/1
  snb_a_ct_errcnt_user_data_in/1 -> sim_out/1
  out_errcnt0/1 -> assert_errcnt0/1
  assert_errcnt0/1 -> reint1/1
  reint1/1 -> concatenate/1
  out_parerrcnt0/1 -> assert_parerrcnt0/1
  assert_parerrcnt0/1 -> reint2/1
  reint2/1 -> concatenate/2
  out_errcnt1/1 -> assert_errcnt1/1
  assert_errcnt1/1 -> reint3/1
  reint3/1 -> concatenate/3
  out_parerrcnt1/1 -> assert_parerrcnt1/1
  assert_parerrcnt1/1 -> reint4/1
  reint4/1 -> concatenate/4
